simulink model "SmaSimulink"  (R2018a)
settings: Solver=FixedStepAuto  StartTime=0.0  StopTime=2  FixedStep=10e-6  RelTol=1e-6
values from neighbouring files (symbols this model uses):
  Af = 80 - ABS_ZERO_TEMP    (= 353.15)    [TempBris.m]    (also in TensileSMA.m = 353)
  As = 70 - ABS_ZERO_TEMP    (= 343.15)    [TempBris.m]    (also in TensileSMA.m = 343)
  Ca = 13.8 * 10^6    (= 13800000)    [TensileSMA.m]
  Cm = 8 * 10^6    (= 8000000)    [TensileSMA.m]
  cSf = 170 * 10^6    (= 170000000)    [TensileSMA.m]
  cSs = 100 * 10^6    (= 100000000)    [TensileSMA.m]
  Da = 6.7 * 10^4 * 10^6    (= 67000000000)    [TensileSMA.m]
  Dm = 2.63 * 10^4 * 10^6    (= 26300000000)    [TensileSMA.m]
  Mf = 40 - ABS_ZERO_TEMP    (= 313.15)    [TempBris.m]    (also in TensileSMA.m = 313)
  Ms = 50 - ABS_ZERO_TEMP    (= 323.15)    [TempBris.m]    (also in TensileSMA.m = 323)
  rEmax = 0.05    [TensileSMA.m]
undefined symbols (not defined in the file or in its folder): martDetwiningStrain, martDetwiningStress, sigma, simout, strain_mart, stress_mart, stressSweep, temp_mart_out
libraries: powerlib_meascontrol x1
(part 1 of 2)
settings Model: Creator=Michau  LastModifiedBy=Michau

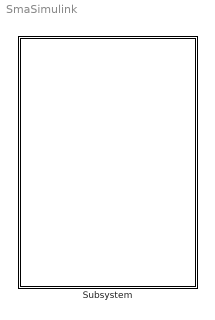
== system SmaSimulink ==
  Subsystem : Subsystem

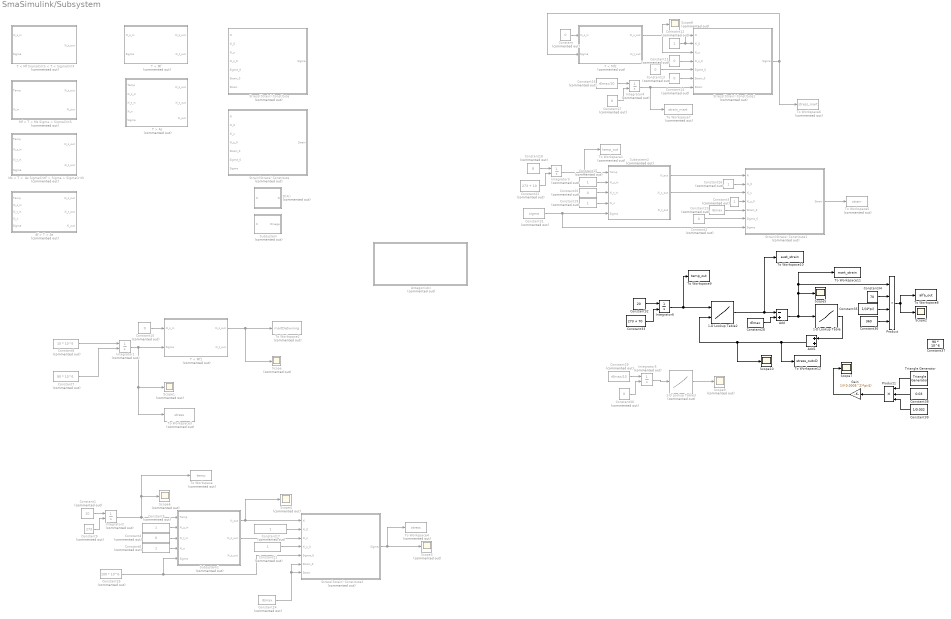
== system SmaSimulink/Subsystem ==
  1-D Lookup Table : Lookup_n-D  NumberOfTableDimensions=1  BreakpointsForDimension1=strain_mart  Table=stress_mart  InternalRulePriority=Speed  RndMeth=Simplest  InputSameDT=on
  1-D Lookup Table2 : Lookup_n-D  BreakpointsForDimension1=temp_mart_out  BreakpointsForDimension2=stressSweep  Table=simout  InternalRulePriority=Speed  RndMeth=Simplest  InputSameDT=on
  1-D Lookup Table3 : Lookup_n-D  Commented=on  NumberOfTableDimensions=1  BreakpointsForDimension1=strain_mart  Table=stress_mart  InternalRulePriority=Speed  RndMeth=Simplest  InputSameDT=on
  Add : Sum  Inputs=-+
  Add1 : Sum
  Af > T > As : Subsystem  Commented=on
  "Antagonistic " : Subsystem  Commented=on
  Constant{,2,4,10..11,13..14,20,27,30} (10 alike) : Constant  Commented=on  Value=0
  Constant1 : Constant  Commented=on  Value=10
  Constant{3,5..6,12,15,17,19,21,26} (9 alike) : Constant  Commented=on
  Constant16 : Constant  Commented=on  Value=rEmax/10
  Constant18 : Constant  Commented=on  Value=8
  Constant22 : Constant  Commented=on  Value=273 + 10
  Constant23 : Constant  Commented=on  Value=rEmax
  Constant24 : Constant  Commented=on  Value=rEmax
  Constant25 : Constant  Commented=on  Value=100 * 10^6
  Constant28 : Constant  Value=rEmax
  Constant29 : Constant  Commented=on  Value=rEmax/10
  Constant31 : Constant  Commented=on  Value=sigma
  Constant32 : Constant  Value=20
  Constant33 : Constant  Value=273 + 70
  Constant34 : Constant  Value=70
  Constant35 : Constant  Value=1/(4*pi)
  Constant36 : Constant  Value=360
  Constant37 : Constant  Value=90 * 10^6
  Constant38 : Constant  Value=0.03
  Constant39 : Constant  Value=1/0.002
  Constant7 : Constant  Commented=on  Value=90 * 10^6
  Constant8 : Constant  Commented=on  Value=10 * 10^6
  Constant9 : Constant  Commented=on  Value=273
  D(Xi) : Subsystem  Commented=on
  Gain : Gain  Gain=1/((0.0005^2)*pi/4)
  Integrator{1..5} (5 alike) : Integrator  Commented=on  InitialConditionSource=external
  Integrator6 : Integrator  InitialConditionSource=external
  Mf < T < Ms Sigma < SigmaCritS : Subsystem  Commented=on
  Ms < T <  As SigmaCritF > Sigma > SigmaCritS : Subsystem  Commented=on
  Product : Product  Inputs=4
  Product1 : Product  Inputs=3
  Scope{,1,3..4,6,8..9} (7 alike) : Scope  Commented=on
  Scope{2,5,7,10} (4 alike) : Scope
  Strain(Stress) Constitute : Subsystem  Commented=on
  Strain(Stress) Constitute1 : Subsystem  Commented=on
  Stress(Strain) Constitute : Subsystem  Commented=on
  Stress(Strain) Constitute1 : Subsystem  Commented=on
  Stress(Strain) Constitute2 : Subsystem  Commented=on
  Subsystem : Subsystem  Commented=on
  Subsystem1 : Subsystem  Commented=on
  Subsystem2 : Subsystem  Commented=on
  T < Mf : Subsystem  Commented=on
  T < Mf SigmaCritS < T < SigmaCritF : Subsystem  Commented=on
  T < Mf1 : Subsystem  Commented=on
  T < Mf2 : Subsystem  Commented=on
  T > As : Subsystem  Commented=on
  To Workspace : ToWorkspace  Commented=on  VariableName=temp  SampleTime=-1
  To Workspace1 : ToWorkspace  Commented=on  VariableName=temp_out  SampleTime=-1
  To Workspace10 : ToWorkspace  VariableName=aust_strain  SampleTime=-1
  To Workspace11 : ToWorkspace  VariableName=mart_strain  SampleTime=-1
  To Workspace12 : ToWorkspace  VariableName=stress_outxD  SampleTime=-1
  To Workspace2 : ToWorkspace  Commented=on  VariableName=martDetwining  SampleTime=-1
  To Workspace3 : ToWorkspace  Commented=on  VariableName=stress  SampleTime=-1
  To Workspace4 : ToWorkspace  Commented=on  VariableName=stress  SampleTime=-1
  To Workspace5 : ToWorkspace  Commented=on  VariableName=strain  SaveFormat=Timeseries  SampleTime=-1
  To Workspace6 : ToWorkspace  Commented=on  VariableName=stress_mart  SampleTime=-1
  To Workspace7 : ToWorkspace  Commented=on  VariableName=strain_mart  SampleTime=-1
  To Workspace8 : ToWorkspace  VariableName=alfa_out  SampleTime=-1
  To Workspace9 : ToWorkspace  VariableName=temp_out  SampleTime=-1
  Triangle Generator : powerlib_meascontrol/Pulse & Signal Generators/Triangle Generator  Freq=1/4  Phase=90  Ts=0
  wires:
  Constant18/1 -> Integrator3/1
  Constant22/1 -> Integrator3/2
  Constant26/1 -> Strain(Stress) Constitute1/2(Xi_0)
  Constant3/1 -> Strain(Stress) Constitute1/4(Xi_s_0)
  ? -> Stress(Strain) Constitute/5(Sigma_0)
  Strain(Stress) Constitute1/1(Strain) -> To Workspace5/1
  Constant5/1 -> Subsystem1/2(Xi_s_in)
  Constant6/1 -> Subsystem1/4(Xi_n)
  Constant9/1 -> Integrator2/2
  Integrator2/1 -> To Workspace/1, Scope6/1, Subsystem1/1(Temp)
  Constant1/1 -> Integrator2/1
  Constant4/1 -> Subsystem1/3(Xi_t_in)
  Constant17/1 -> Stress(Strain) Constitute2/2(Xi_0)
  Subsystem1/1(Xi_out) -> Scope4/1, Stress(Strain) Constitute2/1(Xi)
  Constant21/1 -> Stress(Strain) Constitute2/4(Xi_s_0)
  Subsystem1/2(Xi_s_out) -> Stress(Strain) Constitute2/3(Xi_s)
  Constant24/1 -> Stress(Strain) Constitute2/6(Strain_0), Stress(Strain) Constitute2/7(Strain)
  Constant25/1 -> Subsystem1/5(Sigma), Stress(Strain) Constitute2/5(Sigma_0)
  Stress(Strain) Constitute2/1(Sigma) -> To Workspace4/1, Scope3/1
  Integrator1/1 -> T < Mf1/2(Sigma), Scope1/1, To Workspace3/1
  Constant10/1 -> T < Mf1/1(Xi_s_in)
  T < Mf1/1(Xi_s_out) -> Scope/1, To Workspace2/1
  Constant7/1 -> Integrator1/2
  Constant8/1 -> Integrator1/1
  T < Mf2/1(Xi_s_out) -> Scope8/1, Stress(Strain) Constitute1/3(Xi_s)
  Constant/1 -> T < Mf2/1(Xi_s_in)
  Constant11/1 -> Stress(Strain) Constitute1/4(Xi_s_0)
  Constant12/1 -> Stress(Strain) Constitute1/1(Xi), Stress(Strain) Constitute1/2(Xi_0)
  Constant13/1 -> Stress(Strain) Constitute1/5(Sigma_0)
  Constant14/1 -> Stress(Strain) Constitute1/6(Strain_0)
  Integrator4/1 -> To Workspace7/1, Stress(Strain) Constitute1/7(Strain)
  Constant27/1 -> Integrator4/2
  Constant16/1 -> Integrator4/1
  Stress(Strain) Constitute1/1(Sigma) -> T < Mf2/2(Sigma), To Workspace6/1
  Subsystem2/1(Xi_out) -> Strain(Stress) Constitute1/1(Xi)
  Subsystem2/2(Xi_s_out) -> Strain(Stress) Constitute1/3(Xi_s)
  Integrator3/1 -> To Workspace1/1, Subsystem2/1(Temp)
  Constant15/1 -> Subsystem2/2(Xi_s_in)
  Constant19/1 -> Subsystem2/4(Xi_n)
  Constant20/1 -> Subsystem2/3(Xi_t_in)
  Constant23/1 -> Strain(Stress) Constitute1/5(Strain_0)
  Constant2/1 -> Strain(Stress) Constitute1/6(Sigma_0)
  Constant28/1 -> Add/2
  Add/1 -> Scope5/1, To Workspace11/1, Product/1, 1-D Lookup Table/1
  Constant30/1 -> Integrator5/2
  Integrator5/1 -> 1-D Lookup Table3/1
  Constant29/1 -> Integrator5/1
  1-D Lookup Table3/1 -> Scope9/1
  Constant31/1 -> Strain(Stress) Constitute1/7(Sigma), Subsystem2/5(Sigma)
  Constant33/1 -> Integrator6/2
  Constant32/1 -> Integrator6/1
  Integrator6/1 -> To Workspace9/1, 1-D Lookup Table2/1
  1-D Lookup Table2/1 -> To Workspace10/1, Add/1
  Constant34/1 -> Product/2
  Constant35/1 -> Product/3
  Product/1 -> To Workspace8/1, Scope2/1
  Constant36/1 -> Product/4
  1-D Lookup Table/1 -> Add1/1
  Add1/1 -> To Workspace12/1, Scope10/1, 1-D Lookup Table2/2
  Triangle Generator/1 -> Product1/1
  Constant38/1 -> Product1/2
  Constant39/1 -> Product1/3
  Product1/1 -> Gain/1
  Gain/1 -> Scope7/1

== system SmaSimulink/Subsystem/Af > T > As ==
  Temp : Inport
  Xi_s_in : Inport  Port=2
  Xi_t_in : Inport  Port=3
  Xi_n : Inport  Port=4
  Sigma : Inport  Port=5
  "T > As Xi " : Subsystem
  T > As Xi_s : Subsystem
  T > As Xi_t : Subsystem
  Xi_s_out : Outport
  Xi_t_out : Outport  Port=2
  Xi_out : Outport  Port=3
  wires:
  Sigma/1 -> "T > As Xi "/3("Sigma ")
  "T > As Xi "/1(Xi_out) -> T > As Xi_s/3(Xi_out), T > As Xi_t/3(Xi_out), Xi_out/1
  Xi_s_in/1 -> T > As Xi_s/1("Xi_s_in ")
  Xi_n/1 -> "T > As Xi "/1(Xi_in), T > As Xi_t/2(Xi_in), T > As Xi_s/2(Xi_in)
  T > As Xi_s/1(Xi_s_out) -> Xi_s_out/1
  Temp/1 -> "T > As Xi "/2(T)
  Xi_t_in/1 -> T > As Xi_t/1("Xi_t_in ")
  T > As Xi_t/1(Xi_t_out) -> Xi_t_out/1

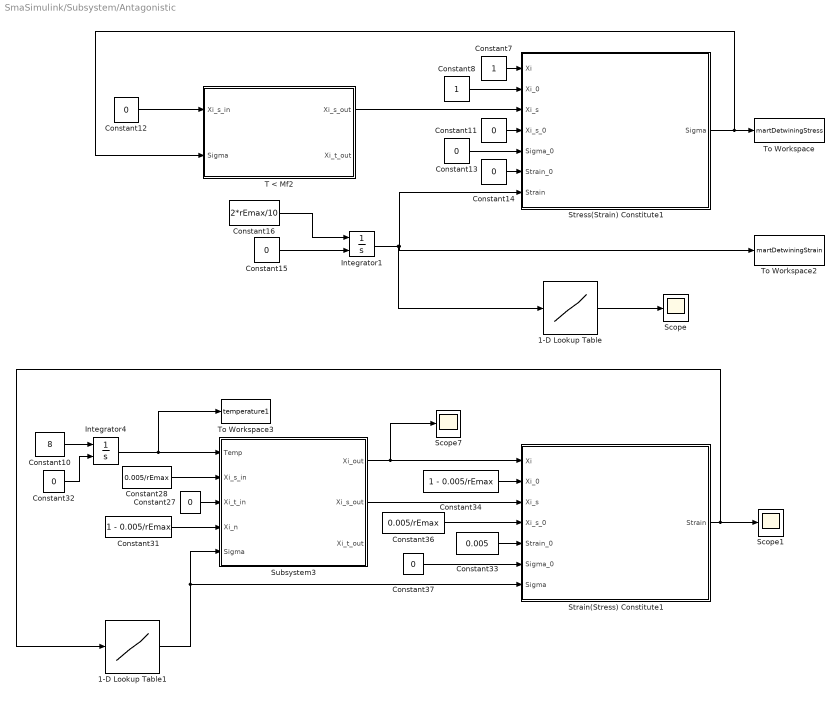
== system SmaSimulink/Subsystem/Antagonistic  ==
  1-D Lookup Table : Lookup_n-D  NumberOfTableDimensions=1  BreakpointsForDimension1=martDetwiningStrain  Table=martDetwiningStress  InternalRulePriority=Speed  RndMeth=Simplest  InputSameDT=on
  1-D Lookup Table1 : Lookup_n-D  NumberOfTableDimensions=1  BreakpointsForDimension1=martDetwiningStrain  Table=martDetwiningStress  InternalRulePriority=Speed  RndMeth=Simplest  InputSameDT=on
  Constant10 : Constant  Value=8
  Constant{11..15,27,32,37} (8 alike) : Constant  Value=0
  Constant16 : Constant  Value=2*rEmax/10
  Constant28 : Constant  Value=0.005/rEmax
  Constant31 : Constant  Value=1 - 0.005/rEmax
  Constant33 : Constant  Value=0.005
  Constant34 : Constant  Value=1 - 0.005/rEmax
  Constant36 : Constant  Value=0.005/rEmax
  Constant7 : Constant
  Constant8 : Constant
  Integrator1 : Integrator  InitialConditionSource=external
  Integrator4 : Integrator  InitialConditionSource=external
  Scope : Scope
  Scope1 : Scope
  Scope7 : Scope
  Strain(Stress) Constitute1 : Subsystem
  Stress(Strain) Constitute1 : Subsystem
  Subsystem3 : Subsystem
  T < Mf2 : Subsystem
  To Workspace : ToWorkspace  VariableName=martDetwiningStress  SampleTime=-1
  To Workspace2 : ToWorkspace  VariableName=martDetwiningStrain  SampleTime=-1
  To Workspace3 : ToWorkspace  VariableName=temperature1  SampleTime=-1
  wires:
  Constant7/1 -> Stress(Strain) Constitute1/1(Xi)
  Stress(Strain) Constitute1/1(Sigma) -> To Workspace/1, T < Mf2/2(Sigma)
  Constant28/1 -> Subsystem3/2(Xi_s_in)
  Constant8/1 -> Stress(Strain) Constitute1/2(Xi_0)
  Constant12/1 -> T < Mf2/1(Xi_s_in)
  Constant34/1 -> Strain(Stress) Constitute1/2(Xi_0)
  Constant16/1 -> Integrator1/1
  Strain(Stress) Constitute1/1(Strain) -> Scope1/1, 1-D Lookup Table1/1
  Integrator4/1 -> To Workspace3/1, Subsystem3/1(Temp)
  Integrator1/1 -> 1-D Lookup Table/1, To Workspace2/1, Stress(Strain) Constitute1/7(Strain)
  Constant14/1 -> Stress(Strain) Constitute1/6(Strain_0)
  T < Mf2/1(Xi_s_out) -> Stress(Strain) Constitute1/3(Xi_s)
  Subsystem3/1(Xi_out) -> Scope7/1, Strain(Stress) Constitute1/1(Xi)
  1-D Lookup Table/1 -> Scope/1
  Constant15/1 -> Integrator1/2
  Constant37/1 -> Strain(Stress) Constitute1/6(Sigma_0)
  Constant33/1 -> Strain(Stress) Constitute1/5(Strain_0)
  Constant32/1 -> Integrator4/2
  Constant31/1 -> Subsystem3/4(Xi_n)
  Constant11/1 -> Stress(Strain) Constitute1/4(Xi_s_0)
  Constant36/1 -> Strain(Stress) Constitute1/4(Xi_s_0)
  Constant10/1 -> Integrator4/1
  Subsystem3/2(Xi_s_out) -> Strain(Stress) Constitute1/3(Xi_s)
  1-D Lookup Table1/1 -> Strain(Stress) Constitute1/7(Sigma), Subsystem3/5(Sigma)
  Constant13/1 -> Stress(Strain) Constitute1/5(Sigma_0)
  Constant27/1 -> Subsystem3/3(Xi_t_in)

== system SmaSimulink/Subsystem/D(Xi) ==
  Xi : Inport
  Add : Sum
  Constant : Constant  Value=Dm-Da
  Constant1 : Constant  Value=Da
  Product : Product
  D : Outport
  wires:
  Xi/1 -> Product/2
  Product/1 -> Add/1
  Constant1/1 -> Add/2
  Constant/1 -> Product/1
  Add/1 -> D/1

== system SmaSimulink/Subsystem/Mf < T < Ms Sigma < SigmaCritS ==
  Temp : Inport
  Xi_in : Inport  Port=2
  Add : Sum  Inputs=-+
  Add1 : Sum  Inputs=+-
  Add2 : Sum
  Constant : Constant
  Constant1 : Constant
  Constant2 : Constant  Value=pi/(Ms-Mf)
  Constant4 : Constant  Value=Mf
  Cos1 : Trigonometry  Operator=cos
  Product1 : Product
  Product3 : Product
  "[(1-x)/2]" : Subsystem
  "Xi_t_out " : Outport
  Xi_out : Outport  Port=2
  wires:
  "[(1-x)/2]"/1(Out) -> Product1/2
  Constant1/1 -> Add2/1
  Xi_in/1 -> "[(1-x)/2]"/1(In)
  Product3/1 -> Cos1/1
  Temp/1 -> Add1/1
  Add1/1 -> Product3/2
  Add2/1 -> Product1/1
  Constant2/1 -> Product3/1
  Cos1/1 -> Add2/2
  Constant4/1 -> Add1/2
  Constant/1 -> Add/2
  Product1/1 -> "Xi_t_out "/1, Add/1
  Add/1 -> Xi_out/1

== system SmaSimulink/Subsystem/Ms < T <  As SigmaCritF > Sigma > SigmaCritS ==
  Temp : Inport
  Xi_s_in : Inport  Port=2
  Xi_t_in : Inport  Port=3
  Sigma : Inport  Port=4
  T > Ms Xi_s : Subsystem
  T > Ms Xi_t : Subsystem
  Xi_s_out : Outport
  Xi_t_out : Outport  Port=2
  wires:
  Sigma/1 -> T > Ms Xi_s/2(Sigma)
  Temp/1 -> T > Ms Xi_s/3(Temp)
  Xi_s_in/1 -> T > Ms Xi_t/2(Xi_s_in), T > Ms Xi_s/1(Xi_s_in)
  Xi_t_in/1 -> T > Ms Xi_t/1(Xi_t_in)
  T > Ms Xi_s/1(Xi_s_out) -> T > Ms Xi_t/3(Xi_s_out), Xi_s_out/1
  T > Ms Xi_t/1(Xi_t_out) -> Xi_t_out/1

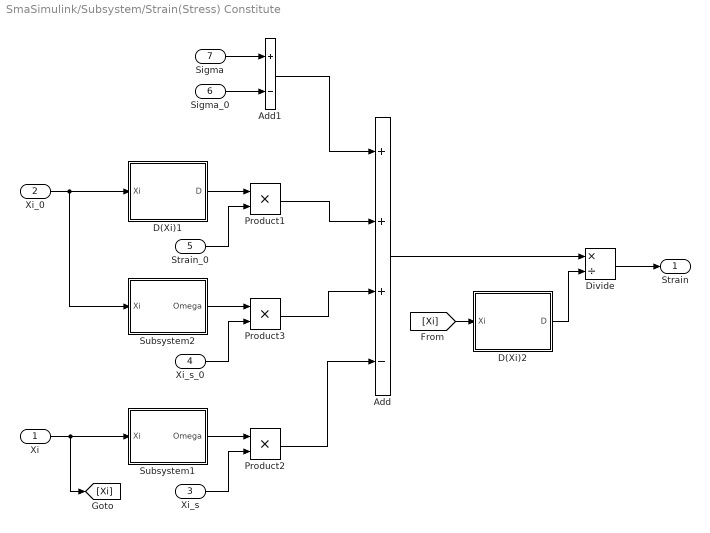
== system SmaSimulink/Subsystem/Strain(Stress) Constitute ==
  Xi : Inport
  Xi_0 : Inport  Port=2
  Xi_s : Inport  Port=3
  Xi_s_0 : Inport  Port=4
  Strain_0 : Inport  Port=5
  Sigma_0 : Inport  Port=6
  Sigma : Inport  Port=7
  Add : Sum  Inputs=+++-
  Add1 : Sum  Inputs=+-
  D(Xi)1 : Subsystem
  D(Xi)2 : Subsystem
  Divide : Product  Inputs=*/
  Product1 : Product
  Product2 : Product
  Product3 : Product
  Subsystem1 : Subsystem
  Subsystem2 : Subsystem
  Strain : Outport
  wires:
  D(Xi)1/1(D) -> Product1/1
  Strain_0/1 -> Product1/2
  Xi/1 -> Subsystem1/1(Xi), [Xi]
  Subsystem1/1(Omega) -> Product2/1
  Xi_0/1 -> Subsystem2/1(Xi), D(Xi)1/1(Xi)
  Subsystem2/1(Omega) -> Product3/1
  Xi_s_0/1 -> Product3/2
  Add/1 -> Divide/1
  Sigma_0/1 -> Add1/2
  Sigma/1 -> Add1/1
  Add1/1 -> Add/1
  Xi_s/1 -> Product2/2
  Product1/1 -> Add/2
  Product3/1 -> Add/3
  Product2/1 -> Add/4
  [Xi] -> D(Xi)2/1(Xi)
  D(Xi)2/1(D) -> Divide/2
  Divide/1 -> Strain/1

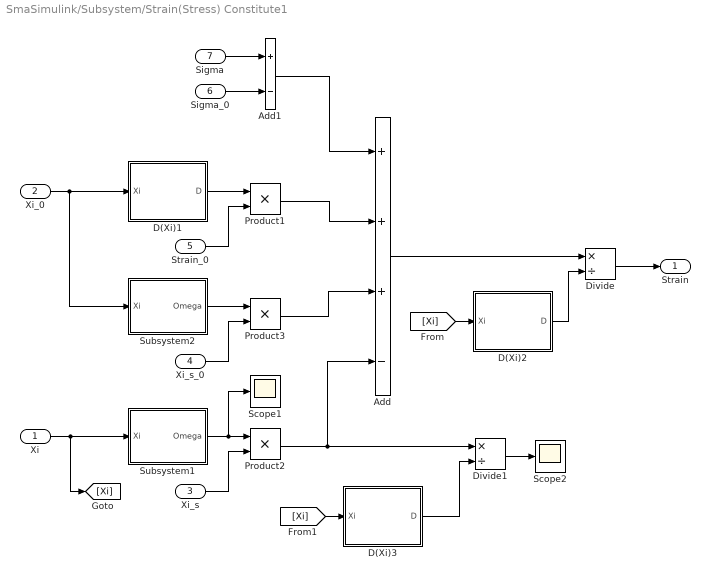
== system SmaSimulink/Subsystem/Strain(Stress) Constitute1 ==
  Xi : Inport
  Xi_0 : Inport  Port=2
  Xi_s : Inport  Port=3
  Xi_s_0 : Inport  Port=4
  Strain_0 : Inport  Port=5
  Sigma_0 : Inport  Port=6
  Sigma : Inport  Port=7
  Add : Sum  Inputs=+++-
  Add1 : Sum  Inputs=+-
  D(Xi)1 : Subsystem
  D(Xi)2 : Subsystem
  D(Xi)3 : Subsystem
  Divide : Product  Inputs=*/
  Divide1 : Product  Inputs=*/
  Product1 : Product
  Product2 : Product
  Product3 : Product
  Scope1 : Scope
  Scope2 : Scope
  Subsystem1 : Subsystem
  Subsystem2 : Subsystem
  Strain : Outport
  wires:
  D(Xi)1/1(D) -> Product1/1
  Strain_0/1 -> Product1/2
  Xi/1 -> Subsystem1/1(Xi), [Xi]
  Subsystem1/1(Omega) -> Scope1/1, Product2/1
  Xi_0/1 -> Subsystem2/1(Xi), D(Xi)1/1(Xi)
  Subsystem2/1(Omega) -> Product3/1
  Xi_s_0/1 -> Product3/2
  Add/1 -> Divide/1
  Sigma_0/1 -> Add1/2
  Sigma/1 -> Add1/1
  Add1/1 -> Add/1
  Xi_s/1 -> Product2/2
  Product1/1 -> Add/2
  Product3/1 -> Add/3
  Product2/1 -> Add/4, Divide1/1
  [Xi] -> D(Xi)2/1(Xi)
  D(Xi)2/1(D) -> Divide/2
  Divide/1 -> Strain/1
  [Xi] -> D(Xi)3/1(Xi)
  D(Xi)3/1(D) -> Divide1/2
  Divide1/1 -> Scope2/1

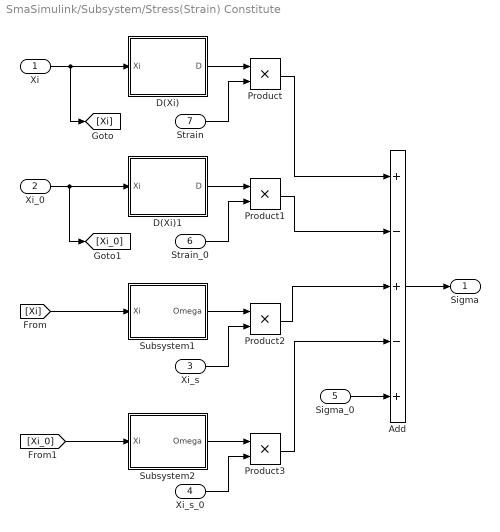
== system SmaSimulink/Subsystem/Stress(Strain) Constitute ==
  Xi : Inport
  Xi_0 : Inport  Port=2
  Xi_s : Inport  Port=3
  Xi_s_0 : Inport  Port=4
  Sigma_0 : Inport  Port=5
  Strain_0 : Inport  Port=6
  Strain : Inport  Port=7
  Add : Sum  Inputs=+-+-+
  D(Xi) : Subsystem
  D(Xi)1 : Subsystem
  Product{,1..3} (4 alike) : Product
  Subsystem1 : Subsystem
  Subsystem2 : Subsystem
  Sigma : Outport
  wires:
  Xi/1 -> [Xi], D(Xi)/1(Xi)
  D(Xi)/1(D) -> Product/1
  Strain/1 -> Product/2
  Xi_0/1 -> [Xi_0], D(Xi)1/1(Xi)
  D(Xi)1/1(D) -> Product1/1
  Strain_0/1 -> Product1/2
  [Xi] -> Subsystem1/1(Xi)
  Subsystem1/1(Omega) -> Product2/1
  Xi_s/1 -> Product2/2
  [Xi_0] -> Subsystem2/1(Xi)
  Subsystem2/1(Omega) -> Product3/1
  Xi_s_0/1 -> Product3/2
  Product/1 -> Add/1
  Product1/1 -> Add/2
  Product2/1 -> Add/3
  Product3/1 -> Add/4
  Sigma_0/1 -> Add/5
  Add/1 -> Sigma/1

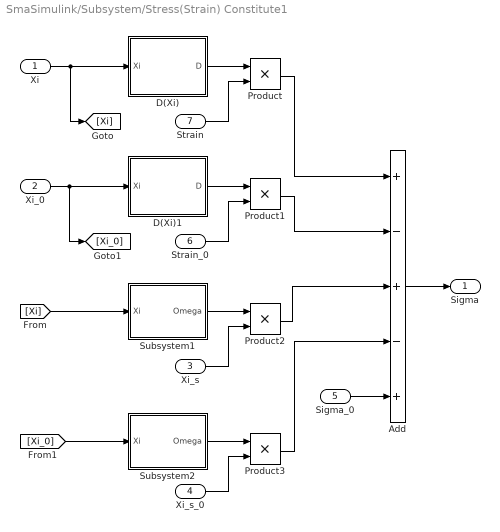
== system SmaSimulink/Subsystem/Stress(Strain) Constitute1 ==
  Xi : Inport
  Xi_0 : Inport  Port=2
  Xi_s : Inport  Port=3
  Xi_s_0 : Inport  Port=4
  Sigma_0 : Inport  Port=5
  Strain_0 : Inport  Port=6
  Strain : Inport  Port=7
  Add : Sum  Inputs=+-+-+
  D(Xi) : Subsystem
  D(Xi)1 : Subsystem
  Product{,1..3} (4 alike) : Product
  Subsystem1 : Subsystem
  Subsystem2 : Subsystem
  Sigma : Outport
  wires:
  Xi/1 -> [Xi], D(Xi)/1(Xi)
  D(Xi)/1(D) -> Product/1
  Strain/1 -> Product/2
  Xi_0/1 -> [Xi_0], D(Xi)1/1(Xi)
  D(Xi)1/1(D) -> Product1/1
  Strain_0/1 -> Product1/2
  [Xi] -> Subsystem1/1(Xi)
  Subsystem1/1(Omega) -> Product2/1
  Xi_s/1 -> Product2/2
  [Xi_0] -> Subsystem2/1(Xi)
  Subsystem2/1(Omega) -> Product3/1
  Xi_s_0/1 -> Product3/2
  Product/1 -> Add/1
  Product1/1 -> Add/2
  Product2/1 -> Add/3
  Product3/1 -> Add/4
  Sigma_0/1 -> Add/5
  Add/1 -> Sigma/1

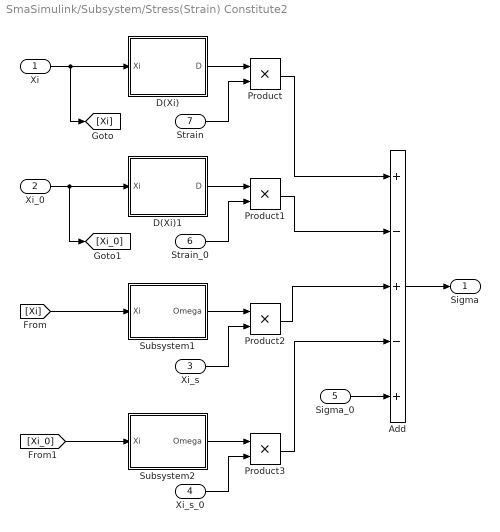
== system SmaSimulink/Subsystem/Stress(Strain) Constitute2 ==
  Xi : Inport
  Xi_0 : Inport  Port=2
  Xi_s : Inport  Port=3
  Xi_s_0 : Inport  Port=4
  Sigma_0 : Inport  Port=5
  Strain_0 : Inport  Port=6
  Strain : Inport  Port=7
  Add : Sum  Inputs=+-+-+
  D(Xi) : Subsystem
  D(Xi)1 : Subsystem
  Product{,1..3} (4 alike) : Product
  Subsystem1 : Subsystem
  Subsystem2 : Subsystem
  Sigma : Outport
  wires:
  Xi/1 -> [Xi], D(Xi)/1(Xi)
  D(Xi)/1(D) -> Product/1
  Strain/1 -> Product/2
  Xi_0/1 -> [Xi_0], D(Xi)1/1(Xi)
  D(Xi)1/1(D) -> Product1/1
  Strain_0/1 -> Product1/2
  [Xi] -> Subsystem1/1(Xi)
  Subsystem1/1(Omega) -> Product2/1
  Xi_s/1 -> Product2/2
  [Xi_0] -> Subsystem2/1(Xi)
  Subsystem2/1(Omega) -> Product3/1
  Xi_s_0/1 -> Product3/2
  Product/1 -> Add/1
  Product1/1 -> Add/2
  Product2/1 -> Add/3
  Product3/1 -> Add/4
  Sigma_0/1 -> Add/5
  Add/1 -> Sigma/1

== system SmaSimulink/Subsystem/Subsystem ==
  Xi : Inport
  Constant : Constant  Value=-rEmax
  Product : Product
  Subsystem1 : Subsystem
  Omega : Outport
  wires:
  Product/1 -> Omega/1
  Subsystem1/1(D) -> Product/1
  Constant/1 -> Product/2
  Xi/1 -> Subsystem1/1(Xi)

== system SmaSimulink/Subsystem/Subsystem1 ==
  Temp : Inport
  Xi_s_in : Inport  Port=2
  Xi_t_in : Inport  Port=3
  Xi_n : Inport  Port=4
  Sigma : Inport  Port=5
  Af > T > As1 : Subsystem
  Demux : Demux  Outputs=3
  Memory : Memory
  Mux : Mux  Inputs=3
  Mux2 : Mux  Inputs=3
  Range check : Subsystem
  Xi_out : Outport
  Xi_s_out : Outport  Port=2
  Xi_t_out : Outport  Port=3
  wires:
  Af > T > As1/2(Xi_t_out) -> Mux/2
  Af > T > As1/3(Xi_out) -> Mux/3
  Sigma/1 -> Memory/1, Af > T > As1/5(Sigma)
  Temp/1 -> Range check/1(T), Af > T > As1/1(Temp)
  Xi_n/1 -> Mux2/3, Af > T > As1/4(Xi_n)
  Xi_s_in/1 -> Mux2/1, Af > T > As1/2(Xi_s_in)
  Xi_t_in/1 -> Mux2/2, Af > T > As1/3(Xi_t_in)
  Af > T > As1/1(Xi_s_out) -> Mux/1
  Demux/1 -> Xi_s_out/1
  Demux/2 -> Xi_t_out/1
  Demux/3 -> Xi_out/1
  Mux/1 -> Range check/2(Xis_new)
  Mux2/1 -> Range check/3(Xis_old)
  Range check/1(Out1) -> Demux/1
  Memory/1 -> Range check/4(Stress)

== system SmaSimulink/Subsystem/Subsystem2 ==
  Temp : Inport
  Xi_s_in : Inport  Port=2
  Xi_t_in : Inport  Port=3
  Xi_n : Inport  Port=4
  Sigma : Inport  Port=5
  Af > T > As1 : Subsystem
  Demux : Demux  Outputs=3
  Memory : Memory
  Mux : Mux  Inputs=3
  Mux2 : Mux  Inputs=3
  Range check : Subsystem
  Xi_out : Outport
  Xi_s_out : Outport  Port=2
  Xi_t_out : Outport  Port=3
  wires:
  Af > T > As1/2(Xi_t_out) -> Mux/2
  Af > T > As1/3(Xi_out) -> Mux/3
  Sigma/1 -> Memory/1, Af > T > As1/5(Sigma)
  Temp/1 -> Range check/1(T), Af > T > As1/1(Temp)
  Xi_n/1 -> Mux2/3, Af > T > As1/4(Xi_n)
  Xi_s_in/1 -> Mux2/1, Af > T > As1/2(Xi_s_in)
  Xi_t_in/1 -> Mux2/2, Af > T > As1/3(Xi_t_in)
  Af > T > As1/1(Xi_s_out) -> Mux/1
  Demux/1 -> Xi_s_out/1
  Demux/2 -> Xi_t_out/1
  Demux/3 -> Xi_out/1
  Mux/1 -> Range check/2(Xis_new)
  Mux2/1 -> Range check/3(Xis_old)
  Range check/1(Out1) -> Demux/1
  Memory/1 -> Range check/4(Stress)

== system SmaSimulink/Subsystem/T < Mf ==
  Xi_s_in : Inport
  Sigma : Inport  Port=2
  Add : Sum  Inputs=-+
  Constant3 : Constant  Value=0
  Constant4 : Constant
  Constant5 : Constant
  Switch : Switch  Criteria=u2 > Threshold  Threshold=cSs
  Switch1 : Switch  Criteria=u2 > Threshold  Threshold=cSf
  T < Mf SigmaCritS < T < SigmaCritF : Subsystem
  Xi_s_out : Outport
  "Xi_t_out " : Outport  Port=2
  wires:
  Constant3/1 -> Switch/3
  Sigma/1 -> Switch/2, Switch1/2, T < Mf SigmaCritS < T < SigmaCritF/2(Sigma)
  Switch/1 -> Switch1/3
  T < Mf SigmaCritS < T < SigmaCritF/1(Xi_t_out) -> Switch/1
  Xi_s_in/1 -> T < Mf SigmaCritS < T < SigmaCritF/1(Xi_s_in)
  Constant4/1 -> Add/2
  Switch1/1 -> Xi_s_out/1, Add/1
  Constant5/1 -> Switch1/1
  Add/1 -> "Xi_t_out "/1

== system SmaSimulink/Subsystem/T < Mf SigmaCritS < T < SigmaCritF ==
  Xi_s_in : Inport
  Sigma : Inport  Port=2
  Add1 : Sum  Inputs=+-
  Add3 : Sum
  Constant1 : Constant  Value=cSf
  Constant2 : Constant  Value=pi/(cSs-cSf)
  Cos : Trigonometry  Operator=cos
  Product2 : Product
  Product3 : Product
  "[(1+x)/2]" : Subsystem
  "[(1-x)/2]" : Subsystem
  Xi_t_out : Outport
  wires:
  Cos/1 -> Product2/2
  Product2/1 -> Add3/2
  Add1/1 -> Product3/2
  Sigma/1 -> Add1/1
  Add3/1 -> Xi_t_out/1
  Xi_s_in/1 -> "[(1+x)/2]"/1(In), "[(1-x)/2]"/1(In)
  Product3/1 -> Cos/1
  "[(1+x)/2]"/1(Out) -> Add3/1
  "[(1-x)/2]"/1(Out) -> Product2/1
  Constant2/1 -> Product3/1
  Constant1/1 -> Add1/2

== system SmaSimulink/Subsystem/T < Mf1 ==
  Xi_s_in : Inport
  Sigma : Inport  Port=2
  Add : Sum  Inputs=-+
  Constant3 : Constant  Value=0
  Constant4 : Constant
  Constant5 : Constant
  Switch : Switch  Criteria=u2 > Threshold  Threshold=cSs
  Switch1 : Switch  Criteria=u2 > Threshold  Threshold=cSf
  T < Mf SigmaCritS < T < SigmaCritF : Subsystem
  Xi_s_out : Outport
  "Xi_t_out " : Outport  Port=2
  wires:
  Constant3/1 -> Switch/3
  Sigma/1 -> Switch/2, Switch1/2, T < Mf SigmaCritS < T < SigmaCritF/2(Sigma)
  Switch/1 -> Switch1/3
  T < Mf SigmaCritS < T < SigmaCritF/1(Xi_t_out) -> Switch/1
  Xi_s_in/1 -> T < Mf SigmaCritS < T < SigmaCritF/1(Xi_s_in)
  Constant4/1 -> Add/2
  Switch1/1 -> Xi_s_out/1, Add/1
  Constant5/1 -> Switch1/1
  Add/1 -> "Xi_t_out "/1

== system SmaSimulink/Subsystem/T < Mf2 ==
  Xi_s_in : Inport
  Sigma : Inport  Port=2
  Add : Sum  Inputs=-+
  Constant3 : Constant  Value=0
  Constant4 : Constant
  Constant5 : Constant
  Switch : Switch  Criteria=u2 > Threshold  Threshold=cSs
  Switch1 : Switch  Criteria=u2 > Threshold  Threshold=cSf
  T < Mf SigmaCritS < T < SigmaCritF : Subsystem
  Xi_s_out : Outport
  "Xi_t_out " : Outport  Port=2
  wires:
  Constant3/1 -> Switch/3
  Sigma/1 -> Switch/2, Switch1/2, T < Mf SigmaCritS < T < SigmaCritF/2(Sigma)
  Switch/1 -> Switch1/3
  T < Mf SigmaCritS < T < SigmaCritF/1(Xi_t_out) -> Switch/1
  Xi_s_in/1 -> T < Mf SigmaCritS < T < SigmaCritF/1(Xi_s_in)
  Constant4/1 -> Add/2
  Switch1/1 -> Xi_s_out/1, Add/1
  Constant5/1 -> Switch1/1
  Add/1 -> "Xi_t_out "/1

== system SmaSimulink/Subsystem/T > As ==
  Temp : Inport
  Xi_s_in : Inport  Port=2
  Xi_t_in : Inport  Port=3
  Xi_n : Inport  Port=4
  Sigma : Inport  Port=5
  Af > T > As1 : Subsystem
  Constant3 : Constant  Value=[0 0 0]
  Demux : Demux  Outputs=3
  Mux : Mux  Inputs=3
  Mux2 : Mux  Inputs=3
  Switch : Switch  Criteria=u2 > Threshold  Threshold=As
  Switch1 : Switch  Criteria=u2 > Threshold  Threshold=Af
  Xi_s_out : Outport
  Xi_t_out : Outport  Port=2
  Xi_out : Outport  Port=3
  wires:
  Constant3/1 -> Switch1/1
  Mux2/1 -> Switch/3
  Af > T > As1/2(Xi_t_out) -> Mux/2
  Switch/1 -> Switch1/3
  Af > T > As1/3(Xi_out) -> Mux/3
  Sigma/1 -> Af > T > As1/5(Sigma)
  Temp/1 -> Switch1/2, Switch/2, Af > T > As1/1(Temp)
  Xi_n/1 -> Mux2/3, Af > T > As1/4(Xi_n)
  Xi_s_in/1 -> Mux2/1, Af > T > As1/2(Xi_s_in)
  Xi_t_in/1 -> Mux2/2, Af > T > As1/3(Xi_t_in)
  Af > T > As1/1(Xi_s_out) -> Mux/1
  Mux/1 -> Switch/1
  Switch1/1 -> Demux/1
  Demux/1 -> Xi_s_out/1
  Demux/2 -> Xi_t_out/1
  Demux/3 -> Xi_out/1

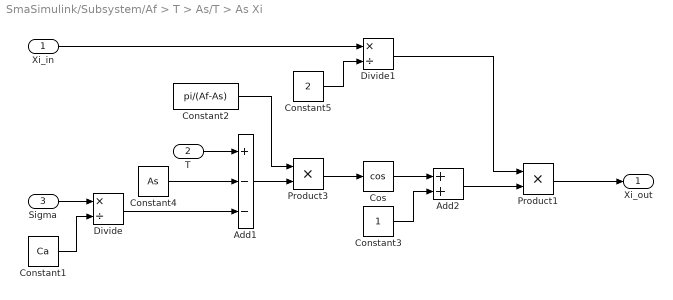
== system SmaSimulink/Subsystem/Af > T > As/T > As Xi  ==
  Xi_in : Inport
  T : Inport  Port=2
  "Sigma " : Inport  Port=3
  Add1 : Sum  Inputs=+--
  Add2 : Sum
  Constant1 : Constant  Value=Ca
  Constant2 : Constant  Value=pi/(Af-As)
  Constant3 : Constant
  Constant4 : Constant  Value=As
  Constant5 : Constant  Value=2
  Cos : Trigonometry  Operator=cos
  Divide : Product  Inputs=*/
  Divide1 : Product  Inputs=*/
  Product1 : Product
  Product3 : Product
  Xi_out : Outport
  wires:
  Constant4/1 -> Add1/2
  Xi_in/1 -> Divide1/1
  T/1 -> Add1/1
  Add1/1 -> Product3/2
  Constant2/1 -> Product3/1
  Product3/1 -> Cos/1
  "Sigma "/1 -> Divide/1
  Constant1/1 -> Divide/2
  Divide/1 -> Add1/3
  Cos/1 -> Add2/1
  Constant3/1 -> Add2/2
  Constant5/1 -> Divide1/2
  Add2/1 -> Product1/2
  Divide1/1 -> Product1/1
  Product1/1 -> Xi_out/1

== system SmaSimulink/Subsystem/Af > T > As/T > As Xi_s ==
  "Xi_s_in " : Inport
  Xi_in : Inport  Port=2
  Xi_out : Inport  Port=3
  Add1 : Sum  Inputs=+-
  Add2 : Sum  Inputs=+-
  Divide : Product  Inputs=*/
  Product1 : Product
  Xi_s_out : Outport
  wires:
  Xi_in/1 -> Add2/1, Divide/2
  "Xi_s_in "/1 -> Add1/1, Divide/1
  Add1/1 -> Xi_s_out/1
  Xi_out/1 -> Add2/2
  Divide/1 -> Product1/1
  Add2/1 -> Product1/2
  Product1/1 -> Add1/2

== system SmaSimulink/Subsystem/Af > T > As/T > As Xi_t ==
  "Xi_t_in " : Inport
  Xi_in : Inport  Port=2
  Xi_out : Inport  Port=3
  Add1 : Sum  Inputs=+-
  Add2 : Sum  Inputs=+-
  Divide : Product  Inputs=*/
  Product1 : Product
  Xi_t_out : Outport
  wires:
  Xi_in/1 -> Add2/1, Divide/2
  "Xi_t_in "/1 -> Add1/1, Divide/1
  Add1/1 -> Xi_t_out/1
  Xi_out/1 -> Add2/2
  Divide/1 -> Product1/1
  Add2/1 -> Product1/2
  Product1/1 -> Add1/2

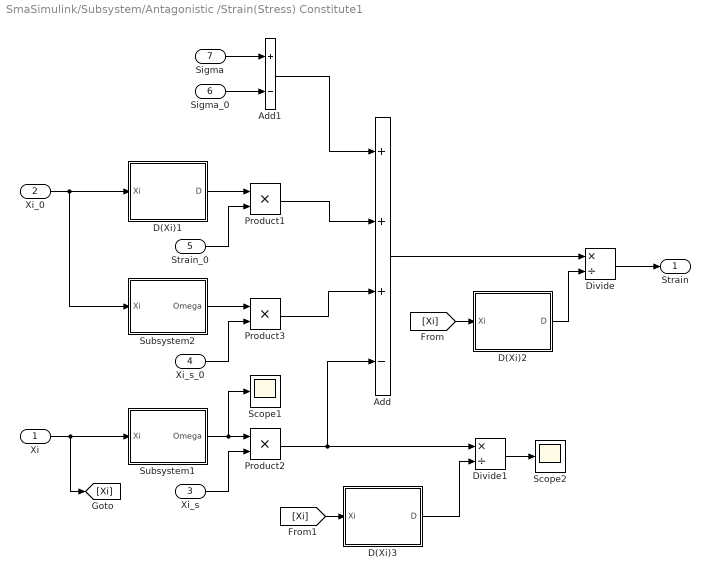
== system SmaSimulink/Subsystem/Antagonistic /Strain(Stress) Constitute1 ==
  Xi : Inport
  Xi_0 : Inport  Port=2
  Xi_s : Inport  Port=3
  Xi_s_0 : Inport  Port=4
  Strain_0 : Inport  Port=5
  Sigma_0 : Inport  Port=6
  Sigma : Inport  Port=7
  Add : Sum  Inputs=+++-
  Add1 : Sum  Inputs=+-
  D(Xi)1 : Subsystem
  D(Xi)2 : Subsystem
  D(Xi)3 : Subsystem
  Divide : Product  Inputs=*/
  Divide1 : Product  Inputs=*/
  Product1 : Product
  Product2 : Product
  Product3 : Product
  Scope1 : Scope
  Scope2 : Scope
  Subsystem1 : Subsystem
  Subsystem2 : Subsystem
  Strain : Outport
  wires:
  D(Xi)1/1(D) -> Product1/1
  Strain_0/1 -> Product1/2
  Xi/1 -> Subsystem1/1(Xi), [Xi]
  Subsystem1/1(Omega) -> Scope1/1, Product2/1
  Xi_0/1 -> Subsystem2/1(Xi), D(Xi)1/1(Xi)
  Subsystem2/1(Omega) -> Product3/1
  Xi_s_0/1 -> Product3/2
  Add/1 -> Divide/1
  Sigma_0/1 -> Add1/2
  Sigma/1 -> Add1/1
  Add1/1 -> Add/1
  Xi_s/1 -> Product2/2
  Product1/1 -> Add/2
  Product3/1 -> Add/3
  Product2/1 -> Add/4, Divide1/1
  [Xi] -> D(Xi)2/1(Xi)
  D(Xi)2/1(D) -> Divide/2
  Divide/1 -> Strain/1
  [Xi] -> D(Xi)3/1(Xi)
  D(Xi)3/1(D) -> Divide1/2
  Divide1/1 -> Scope2/1

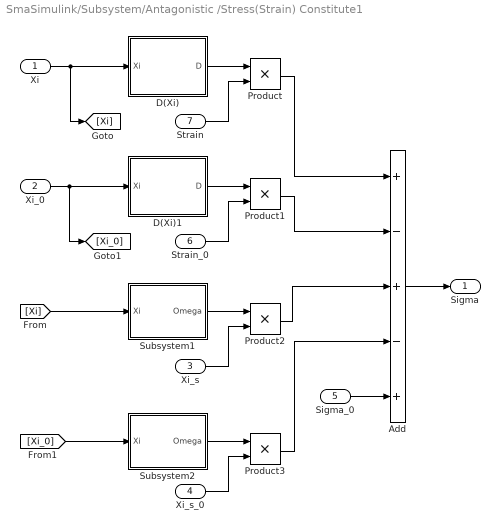
== system SmaSimulink/Subsystem/Antagonistic /Stress(Strain) Constitute1 ==
  Xi : Inport
  Xi_0 : Inport  Port=2
  Xi_s : Inport  Port=3
  Xi_s_0 : Inport  Port=4
  Sigma_0 : Inport  Port=5
  Strain_0 : Inport  Port=6
  Strain : Inport  Port=7
  Add : Sum  Inputs=+-+-+
  D(Xi) : Subsystem
  D(Xi)1 : Subsystem
  Product{,1..3} (4 alike) : Product
  Subsystem1 : Subsystem
  Subsystem2 : Subsystem
  Sigma : Outport
  wires:
  Xi/1 -> [Xi], D(Xi)/1(Xi)
  D(Xi)/1(D) -> Product/1
  Strain/1 -> Product/2
  Xi_0/1 -> [Xi_0], D(Xi)1/1(Xi)
  D(Xi)1/1(D) -> Product1/1
  Strain_0/1 -> Product1/2
  [Xi] -> Subsystem1/1(Xi)
  Subsystem1/1(Omega) -> Product2/1
  Xi_s/1 -> Product2/2
  [Xi_0] -> Subsystem2/1(Xi)
  Subsystem2/1(Omega) -> Product3/1
  Xi_s_0/1 -> Product3/2
  Product/1 -> Add/1
  Product1/1 -> Add/2
  Product2/1 -> Add/3
  Product3/1 -> Add/4
  Sigma_0/1 -> Add/5
  Add/1 -> Sigma/1

== system SmaSimulink/Subsystem/Antagonistic /Subsystem3 ==
  Temp : Inport
  Xi_s_in : Inport  Port=2
  Xi_t_in : Inport  Port=3
  Xi_n : Inport  Port=4
  Sigma : Inport  Port=5
  Af > T > As1 : Subsystem
  Demux : Demux  Outputs=3
  Memory : Memory
  Mux : Mux  Inputs=3
  Mux2 : Mux  Inputs=3
  Range check : Subsystem
  Xi_out : Outport
  Xi_s_out : Outport  Port=2
  Xi_t_out : Outport  Port=3
  wires:
  Af > T > As1/2(Xi_t_out) -> Mux/2
  Af > T > As1/3(Xi_out) -> Mux/3
  Sigma/1 -> Memory/1, Af > T > As1/5(Sigma)
  Temp/1 -> Range check/1(T), Af > T > As1/1(Temp)
  Xi_n/1 -> Mux2/3, Af > T > As1/4(Xi_n)
  Xi_s_in/1 -> Mux2/1, Af > T > As1/2(Xi_s_in)
  Xi_t_in/1 -> Mux2/2, Af > T > As1/3(Xi_t_in)
  Af > T > As1/1(Xi_s_out) -> Mux/1
  Demux/1 -> Xi_s_out/1
  Demux/2 -> Xi_t_out/1
  Demux/3 -> Xi_out/1
  Mux/1 -> Range check/2(Xis_new)
  Mux2/1 -> Range check/3(Xis_old)
  Range check/1(Out1) -> Demux/1
  Memory/1 -> Range check/4(Stress)

== system SmaSimulink/Subsystem/Antagonistic /T < Mf2 ==
  Xi_s_in : Inport
  Sigma : Inport  Port=2
  Add : Sum  Inputs=-+
  Constant3 : Constant  Value=0
  Constant4 : Constant
  Constant5 : Constant
  Switch : Switch  Criteria=u2 > Threshold  Threshold=cSs
  Switch1 : Switch  Criteria=u2 > Threshold  Threshold=cSf
  T < Mf SigmaCritS < T < SigmaCritF : Subsystem
  Xi_s_out : Outport
  "Xi_t_out " : Outport  Port=2
  wires:
  Constant3/1 -> Switch/3
  Sigma/1 -> Switch/2, Switch1/2, T < Mf SigmaCritS < T < SigmaCritF/2(Sigma)
  Switch/1 -> Switch1/3
  T < Mf SigmaCritS < T < SigmaCritF/1(Xi_t_out) -> Switch/1
  Xi_s_in/1 -> T < Mf SigmaCritS < T < SigmaCritF/1(Xi_s_in)
  Constant4/1 -> Add/2
  Switch1/1 -> Xi_s_out/1, Add/1
  Constant5/1 -> Switch1/1
  Add/1 -> "Xi_t_out "/1

== system SmaSimulink/Subsystem/Mf < T < Ms Sigma < SigmaCritS/[(1-x)//2] ==
  In : Inport
  Add1 : Sum  Inputs=+-
  Constant1 : Constant
  Constant3 : Constant  Value=2
  Divide1 : Product  Inputs=*/
  Out : Outport
  wires:
  Constant3/1 -> Divide1/2
  Divide1/1 -> Out/1
  Constant1/1 -> Add1/1
  In/1 -> Add1/2
  Add1/1 -> Divide1/1

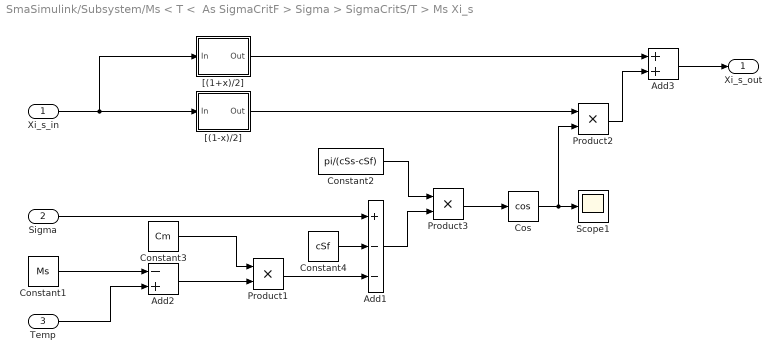
== system SmaSimulink/Subsystem/Ms < T <  As SigmaCritF > Sigma > SigmaCritS/T > Ms Xi_s ==
  Xi_s_in : Inport
  Sigma : Inport  Port=2
  Temp : Inport  Port=3
  Add1 : Sum  Inputs=+--
  Add2 : Sum  Inputs=-+
  Add3 : Sum
  Constant1 : Constant  Value=Ms
  Constant2 : Constant  Value=pi/(cSs-cSf)
  Constant3 : Constant  Value=Cm
  Constant4 : Constant  Value=cSf
  Cos : Trigonometry  Operator=cos
  Product1 : Product
  Product2 : Product
  Product3 : Product
  Scope1 : Scope
  "[(1+x)/2]" : Subsystem
  "[(1-x)/2]" : Subsystem
  Xi_s_out : Outport
  wires:
  Constant4/1 -> Add1/2
  Product1/1 -> Add1/3
  Xi_s_in/1 -> "[(1+x)/2]"/1(In), "[(1-x)/2]"/1(In)
  Add2/1 -> Product1/2
  "[(1+x)/2]"/1(Out) -> Add3/1
  Temp/1 -> Add2/2
  Product2/1 -> Add3/2
  Constant3/1 -> Product1/1
  "[(1-x)/2]"/1(Out) -> Product2/1
  Add3/1 -> Xi_s_out/1
  Constant1/1 -> Add2/1
  Sigma/1 -> Add1/1
  Add1/1 -> Product3/2
  Constant2/1 -> Product3/1
  Product3/1 -> Cos/1
  Cos/1 -> Product2/2, Scope1/1

== system SmaSimulink/Subsystem/Ms < T <  As SigmaCritF > Sigma > SigmaCritS/T > Ms Xi_t ==
  Xi_t_in : Inport
  Xi_s_in : Inport  Port=2
  Xi_s_out : Inport  Port=3
  Add1 : Sum  Inputs=+-
  Add2 : Sum  Inputs=+-
  Add3 : Sum  Inputs=-+
  Constant3 : Constant
  Divide : Product  Inputs=*/
  Product2 : Product
  Xi_t_out : Outport
  wires:
  Product2/1 -> Add1/2
  Add3/1 -> Product2/2
  Xi_s_out/1 -> Add3/2
  Xi_t_in/1 -> Divide/1, Add1/1
  Xi_s_in/1 -> Add3/1, Add2/2
  Add2/1 -> Divide/2
  Constant3/1 -> Add2/1
  Divide/1 -> Product2/1
  Add1/1 -> Xi_t_out/1

== system SmaSimulink/Subsystem/Strain(Stress) Constitute/D(Xi)1 ==
  Xi : Inport
  Add : Sum
  Constant : Constant  Value=Dm-Da
  Constant1 : Constant  Value=Da
  Product : Product
  D : Outport
  wires:
  Xi/1 -> Product/2
  Product/1 -> Add/1
  Constant1/1 -> Add/2
  Constant/1 -> Product/1
  Add/1 -> D/1

== system SmaSimulink/Subsystem/Strain(Stress) Constitute/D(Xi)2 ==
  Xi : Inport
  Add : Sum
  Constant : Constant  Value=Dm-Da
  Constant1 : Constant  Value=Da
  Product : Product
  D : Outport
  wires:
  Xi/1 -> Product/2
  Product/1 -> Add/1
  Constant1/1 -> Add/2
  Constant/1 -> Product/1
  Add/1 -> D/1

== system SmaSimulink/Subsystem/Strain(Stress) Constitute/Subsystem1 ==
  Xi : Inport
  Constant : Constant  Value=-rEmax
  Product : Product
  Subsystem1 : Subsystem
  Omega : Outport
  wires:
  Product/1 -> Omega/1
  Subsystem1/1(D) -> Product/1
  Constant/1 -> Product/2
  Xi/1 -> Subsystem1/1(Xi)

== system SmaSimulink/Subsystem/Strain(Stress) Constitute/Subsystem2 ==
  Xi : Inport
  Constant : Constant  Value=-rEmax
  Product : Product
  Subsystem1 : Subsystem
  Omega : Outport
  wires:
  Product/1 -> Omega/1
  Subsystem1/1(D) -> Product/1
  Constant/1 -> Product/2
  Xi/1 -> Subsystem1/1(Xi)

== system SmaSimulink/Subsystem/Strain(Stress) Constitute1/D(Xi)1 ==
  Xi : Inport
  Add : Sum
  Constant : Constant  Value=Dm-Da
  Constant1 : Constant  Value=Da
  Product : Product
  D : Outport
  wires:
  Xi/1 -> Product/2
  Product/1 -> Add/1
  Constant1/1 -> Add/2
  Constant/1 -> Product/1
  Add/1 -> D/1

== system SmaSimulink/Subsystem/Strain(Stress) Constitute1/D(Xi)2 ==
  Xi : Inport
  Add : Sum
  Constant : Constant  Value=Dm-Da
  Constant1 : Constant  Value=Da
  Product : Product
  D : Outport
  wires:
  Xi/1 -> Product/2
  Product/1 -> Add/1
  Constant1/1 -> Add/2
  Constant/1 -> Product/1
  Add/1 -> D/1

== system SmaSimulink/Subsystem/Strain(Stress) Constitute1/D(Xi)3 ==
  Xi : Inport
  Add : Sum
  Constant : Constant  Value=Dm-Da
  Constant1 : Constant  Value=Da
  Product : Product
  D : Outport
  wires:
  Xi/1 -> Product/2
  Product/1 -> Add/1
  Constant1/1 -> Add/2
  Constant/1 -> Product/1
  Add/1 -> D/1

== system SmaSimulink/Subsystem/Strain(Stress) Constitute1/Subsystem1 ==
  Xi : Inport
  Constant : Constant  Value=-rEmax
  Product : Product
  Subsystem1 : Subsystem
  Omega : Outport
  wires:
  Product/1 -> Omega/1
  Subsystem1/1(D) -> Product/1
  Constant/1 -> Product/2
  Xi/1 -> Subsystem1/1(Xi)

== system SmaSimulink/Subsystem/Strain(Stress) Constitute1/Subsystem2 ==
  Xi : Inport
  Constant : Constant  Value=-rEmax
  Product : Product
  Subsystem1 : Subsystem
  Omega : Outport
  wires:
  Product/1 -> Omega/1
  Subsystem1/1(D) -> Product/1
  Constant/1 -> Product/2
  Xi/1 -> Subsystem1/1(Xi)

== system SmaSimulink/Subsystem/Stress(Strain) Constitute/D(Xi) ==
  Xi : Inport
  Add : Sum
  Constant : Constant  Value=Dm-Da
  Constant1 : Constant  Value=Da
  Product : Product
  D : Outport
  wires:
  Xi/1 -> Product/2
  Product/1 -> Add/1
  Constant1/1 -> Add/2
  Constant/1 -> Product/1
  Add/1 -> D/1

== system SmaSimulink/Subsystem/Stress(Strain) Constitute/D(Xi)1 ==
  Xi : Inport
  Add : Sum
  Constant : Constant  Value=Dm-Da
  Constant1 : Constant  Value=Da
  Product : Product
  D : Outport
  wires:
  Xi/1 -> Product/2
  Product/1 -> Add/1
  Constant1/1 -> Add/2
  Constant/1 -> Product/1
  Add/1 -> D/1

== system SmaSimulink/Subsystem/Stress(Strain) Constitute/Subsystem1 ==
  Xi : Inport
  Constant : Constant  Value=-rEmax
  Product : Product
  Subsystem1 : Subsystem
  Omega : Outport
  wires:
  Product/1 -> Omega/1
  Subsystem1/1(D) -> Product/1
  Constant/1 -> Product/2
  Xi/1 -> Subsystem1/1(Xi)

== system SmaSimulink/Subsystem/Stress(Strain) Constitute/Subsystem2 ==
  Xi : Inport
  Constant : Constant  Value=-rEmax
  Product : Product
  Subsystem1 : Subsystem
  Omega : Outport
  wires:
  Product/1 -> Omega/1
  Subsystem1/1(D) -> Product/1
  Constant/1 -> Product/2
  Xi/1 -> Subsystem1/1(Xi)

== system SmaSimulink/Subsystem/Stress(Strain) Constitute1/D(Xi) ==
  Xi : Inport
  Add : Sum
  Constant : Constant  Value=Dm-Da
  Constant1 : Constant  Value=Da
  Product : Product
  D : Outport
  wires:
  Xi/1 -> Product/2
  Product/1 -> Add/1
  Constant1/1 -> Add/2
  Constant/1 -> Product/1
  Add/1 -> D/1

== system SmaSimulink/Subsystem/Stress(Strain) Constitute1/D(Xi)1 ==
  Xi : Inport
  Add : Sum
  Constant : Constant  Value=Dm-Da
  Constant1 : Constant  Value=Da
  Product : Product
  D : Outport
  wires:
  Xi/1 -> Product/2
  Product/1 -> Add/1
  Constant1/1 -> Add/2
  Constant/1 -> Product/1
  Add/1 -> D/1

== system SmaSimulink/Subsystem/Stress(Strain) Constitute1/Subsystem1 ==
  Xi : Inport
  Constant : Constant  Value=-rEmax
  Product : Product
  Subsystem1 : Subsystem
  Omega : Outport
  wires:
  Product/1 -> Omega/1
  Subsystem1/1(D) -> Product/1
  Constant/1 -> Product/2
  Xi/1 -> Subsystem1/1(Xi)

== system SmaSimulink/Subsystem/Stress(Strain) Constitute1/Subsystem2 ==
  Xi : Inport
  Constant : Constant  Value=-rEmax
  Product : Product
  Subsystem1 : Subsystem
  Omega : Outport
  wires:
  Product/1 -> Omega/1
  Subsystem1/1(D) -> Product/1
  Constant/1 -> Product/2
  Xi/1 -> Subsystem1/1(Xi)

== system SmaSimulink/Subsystem/Stress(Strain) Constitute2/D(Xi) ==
  Xi : Inport
  Add : Sum
  Constant : Constant  Value=Dm-Da
  Constant1 : Constant  Value=Da
  Product : Product
  D : Outport
  wires:
  Xi/1 -> Product/2
  Product/1 -> Add/1
  Constant1/1 -> Add/2
  Constant/1 -> Product/1
  Add/1 -> D/1

== system SmaSimulink/Subsystem/Stress(Strain) Constitute2/D(Xi)1 ==
  Xi : Inport
  Add : Sum
  Constant : Constant  Value=Dm-Da
  Constant1 : Constant  Value=Da
  Product : Product
  D : Outport
  wires:
  Xi/1 -> Product/2
  Product/1 -> Add/1
  Constant1/1 -> Add/2
  Constant/1 -> Product/1
  Add/1 -> D/1

== system SmaSimulink/Subsystem/Stress(Strain) Constitute2/Subsystem1 ==
  Xi : Inport
  Constant : Constant  Value=-rEmax
  Product : Product
  Subsystem1 : Subsystem
  Omega : Outport
  wires:
  Product/1 -> Omega/1
  Subsystem1/1(D) -> Product/1
  Constant/1 -> Product/2
  Xi/1 -> Subsystem1/1(Xi)

== system SmaSimulink/Subsystem/Stress(Strain) Constitute2/Subsystem2 ==
  Xi : Inport
  Constant : Constant  Value=-rEmax
  Product : Product
  Subsystem1 : Subsystem
  Omega : Outport
  wires:
  Product/1 -> Omega/1
  Subsystem1/1(D) -> Product/1
  Constant/1 -> Product/2
  Xi/1 -> Subsystem1/1(Xi)

== system SmaSimulink/Subsystem/Subsystem/Subsystem1 ==
  Xi : Inport
  Add : Sum
  Constant : Constant  Value=Dm-Da
  Constant1 : Constant  Value=Da
  Product : Product
  D : Outport
  wires:
  Xi/1 -> Product/2
  Product/1 -> Add/1
  Constant1/1 -> Add/2
  Constant/1 -> Product/1
  Add/1 -> D/1

== system SmaSimulink/Subsystem/Subsystem1/Af > T > As1 ==
  Temp : Inport
  Xi_s_in : Inport  Port=2
  Xi_t_in : Inport  Port=3
  Xi_n : Inport  Port=4
  Sigma : Inport  Port=5
  "T > As Xi " : Subsystem
  T > As Xi_s : Subsystem
  T > As Xi_t : Subsystem
  Xi_s_out : Outport
  Xi_t_out : Outport  Port=2
  Xi_out : Outport  Port=3
  wires:
  Sigma/1 -> "T > As Xi "/3("Sigma ")
  "T > As Xi "/1(Xi_out) -> T > As Xi_s/3(Xi_out), T > As Xi_t/3(Xi_out), Xi_out/1
  Xi_s_in/1 -> T > As Xi_s/1("Xi_s_in ")
  Xi_n/1 -> "T > As Xi "/1(Xi_in), T > As Xi_t/2(Xi_in), T > As Xi_s/2(Xi_in)
  T > As Xi_s/1(Xi_s_out) -> Xi_s_out/1
  Temp/1 -> "T > As Xi "/2(T)
  Xi_t_in/1 -> T > As Xi_t/1("Xi_t_in ")
  T > As Xi_t/1(Xi_t_out) -> Xi_t_out/1

== system SmaSimulink/Subsystem/Subsystem1/Range check ==
  T : Inport
  Xis_new : Inport  Port=2
  Xis_old : Inport  Port=3
  Stress : Inport  Port=4
  Add : Sum  Inputs=-+
  Constant1 : Constant  Value=Ca
  Constant3 : Constant  Value=[0 0 0]
  Divide : Product  Inputs=*/
  Switch : Switch  Criteria=u2 > Threshold  Threshold=As
  Switch1 : Switch  Criteria=u2 > Threshold  Threshold=Af
  Out1 : Outport
  wires:
  Switch/1 -> Switch1/3
  Constant3/1 -> Switch1/1
  Xis_old/1 -> Switch/3
  T/1 -> Add/2
  Xis_new/1 -> Switch/1
  Switch1/1 -> Out1/1
  Add/1 -> Switch/2, Switch1/2
  Stress/1 -> Divide/1
  Constant1/1 -> Divide/2
  Divide/1 -> Add/1

== system SmaSimulink/Subsystem/Subsystem2/Af > T > As1 ==
  Temp : Inport
  Xi_s_in : Inport  Port=2
  Xi_t_in : Inport  Port=3
  Xi_n : Inport  Port=4
  Sigma : Inport  Port=5
  "T > As Xi " : Subsystem
  T > As Xi_s : Subsystem
  T > As Xi_t : Subsystem
  Xi_s_out : Outport
  Xi_t_out : Outport  Port=2
  Xi_out : Outport  Port=3
  wires:
  Sigma/1 -> "T > As Xi "/3("Sigma ")
  "T > As Xi "/1(Xi_out) -> T > As Xi_s/3(Xi_out), T > As Xi_t/3(Xi_out), Xi_out/1
  Xi_s_in/1 -> T > As Xi_s/1("Xi_s_in ")
  Xi_n/1 -> "T > As Xi "/1(Xi_in), T > As Xi_t/2(Xi_in), T > As Xi_s/2(Xi_in)
  T > As Xi_s/1(Xi_s_out) -> Xi_s_out/1
  Temp/1 -> "T > As Xi "/2(T)
  Xi_t_in/1 -> T > As Xi_t/1("Xi_t_in ")
  T > As Xi_t/1(Xi_t_out) -> Xi_t_out/1

== system SmaSimulink/Subsystem/Subsystem2/Range check ==
  T : Inport
  Xis_new : Inport  Port=2
  Xis_old : Inport  Port=3
  Stress : Inport  Port=4
  Add : Sum  Inputs=-+
  Constant1 : Constant  Value=Ca
  Constant3 : Constant  Value=[0 0 0]
  Divide : Product  Inputs=*/
  Switch : Switch  Criteria=u2 > Threshold  Threshold=As
  Switch1 : Switch  Criteria=u2 > Threshold  Threshold=Af
  Out1 : Outport
  wires:
  Switch/1 -> Switch1/3
  Constant3/1 -> Switch1/1
  Xis_old/1 -> Switch/3
  T/1 -> Add/2
  Xis_new/1 -> Switch/1
  Switch1/1 -> Out1/1
  Add/1 -> Switch/2, Switch1/2
  Stress/1 -> Divide/1
  Constant1/1 -> Divide/2
  Divide/1 -> Add/1

== system SmaSimulink/Subsystem/T < Mf/T < Mf SigmaCritS < T < SigmaCritF ==
  Xi_s_in : Inport
  Sigma : Inport  Port=2
  Add1 : Sum  Inputs=+-
  Add3 : Sum
  Constant1 : Constant  Value=cSf
  Constant2 : Constant  Value=pi/(cSs-cSf)
  Cos : Trigonometry  Operator=cos
  Product2 : Product
  Product3 : Product
  "[(1+x)/2]" : Subsystem
  "[(1-x)/2]" : Subsystem
  Xi_t_out : Outport
  wires:
  Cos/1 -> Product2/2
  Product2/1 -> Add3/2
  Add1/1 -> Product3/2
  Sigma/1 -> Add1/1
  Add3/1 -> Xi_t_out/1
  Xi_s_in/1 -> "[(1+x)/2]"/1(In), "[(1-x)/2]"/1(In)
  Product3/1 -> Cos/1
  "[(1+x)/2]"/1(Out) -> Add3/1
  "[(1-x)/2]"/1(Out) -> Product2/1
  Constant2/1 -> Product3/1
  Constant1/1 -> Add1/2

== system SmaSimulink/Subsystem/T < Mf SigmaCritS < T < SigmaCritF/[(1+x)//2] ==
  In : Inport
  Add1 : Sum
  Constant1 : Constant
  Constant3 : Constant  Value=2
  Divide1 : Product  Inputs=*/
  Out : Outport
  wires:
  Constant3/1 -> Divide1/2
  Divide1/1 -> Out/1
  Constant1/1 -> Add1/1
  In/1 -> Add1/2
  Add1/1 -> Divide1/1

== system SmaSimulink/Subsystem/T < Mf SigmaCritS < T < SigmaCritF/[(1-x)//2] ==
  In : Inport
  Add1 : Sum  Inputs=+-
  Constant1 : Constant
  Constant3 : Constant  Value=2
  Divide1 : Product  Inputs=*/
  Out : Outport
  wires:
  Constant3/1 -> Divide1/2
  Divide1/1 -> Out/1
  Constant1/1 -> Add1/1
  In/1 -> Add1/2
  Add1/1 -> Divide1/1

== system SmaSimulink/Subsystem/T < Mf1/T < Mf SigmaCritS < T < SigmaCritF ==
  Xi_s_in : Inport
  Sigma : Inport  Port=2
  Add1 : Sum  Inputs=+-
  Add3 : Sum
  Constant1 : Constant  Value=cSf
  Constant2 : Constant  Value=pi/(cSs-cSf)
  Cos : Trigonometry  Operator=cos
  Product2 : Product
  Product3 : Product
  "[(1+x)/2]" : Subsystem
  "[(1-x)/2]" : Subsystem
  Xi_t_out : Outport
  wires:
  Cos/1 -> Product2/2
  Product2/1 -> Add3/2
  Add1/1 -> Product3/2
  Sigma/1 -> Add1/1
  Add3/1 -> Xi_t_out/1
  Xi_s_in/1 -> "[(1+x)/2]"/1(In), "[(1-x)/2]"/1(In)
  Product3/1 -> Cos/1
  "[(1+x)/2]"/1(Out) -> Add3/1
  "[(1-x)/2]"/1(Out) -> Product2/1
  Constant2/1 -> Product3/1
  Constant1/1 -> Add1/2

== system SmaSimulink/Subsystem/T < Mf2/T < Mf SigmaCritS < T < SigmaCritF ==
  Xi_s_in : Inport
  Sigma : Inport  Port=2
  Add1 : Sum  Inputs=+-
  Add3 : Sum
  Constant1 : Constant  Value=cSf
  Constant2 : Constant  Value=pi/(cSs-cSf)
  Cos : Trigonometry  Operator=cos
  Product2 : Product
  Product3 : Product
  "[(1+x)/2]" : Subsystem
  "[(1-x)/2]" : Subsystem
  Xi_t_out : Outport
  wires:
  Cos/1 -> Product2/2
  Product2/1 -> Add3/2
  Add1/1 -> Product3/2
  Sigma/1 -> Add1/1
  Add3/1 -> Xi_t_out/1
  Xi_s_in/1 -> "[(1+x)/2]"/1(In), "[(1-x)/2]"/1(In)
  Product3/1 -> Cos/1
  "[(1+x)/2]"/1(Out) -> Add3/1
  "[(1-x)/2]"/1(Out) -> Product2/1
  Constant2/1 -> Product3/1
  Constant1/1 -> Add1/2

== system SmaSimulink/Subsystem/T > As/Af > T > As1 ==
  Temp : Inport
  Xi_s_in : Inport  Port=2
  Xi_t_in : Inport  Port=3
  Xi_n : Inport  Port=4
  Sigma : Inport  Port=5
  "T > As Xi " : Subsystem
  T > As Xi_s : Subsystem
  T > As Xi_t : Subsystem
  Xi_s_out : Outport
  Xi_t_out : Outport  Port=2
  Xi_out : Outport  Port=3
  wires:
  Sigma/1 -> "T > As Xi "/3("Sigma ")
  "T > As Xi "/1(Xi_out) -> T > As Xi_s/3(Xi_out), T > As Xi_t/3(Xi_out), Xi_out/1
  Xi_s_in/1 -> T > As Xi_s/1("Xi_s_in ")
  Xi_n/1 -> "T > As Xi "/1(Xi_in), T > As Xi_t/2(Xi_in), T > As Xi_s/2(Xi_in)
  T > As Xi_s/1(Xi_s_out) -> Xi_s_out/1
  Temp/1 -> "T > As Xi "/2(T)
  Xi_t_in/1 -> T > As Xi_t/1("Xi_t_in ")
  T > As Xi_t/1(Xi_t_out) -> Xi_t_out/1

== system SmaSimulink/Subsystem/Antagonistic /Strain(Stress) Constitute1/D(Xi)1 ==
  Xi : Inport
  Add : Sum
  Constant : Constant  Value=Dm-Da
  Constant1 : Constant  Value=Da
  Product : Product
  D : Outport
  wires:
  Xi/1 -> Product/2
  Product/1 -> Add/1
  Constant1/1 -> Add/2
  Constant/1 -> Product/1
  Add/1 -> D/1

== system SmaSimulink/Subsystem/Antagonistic /Strain(Stress) Constitute1/D(Xi)2 ==
  Xi : Inport
  Add : Sum
  Constant : Constant  Value=Dm-Da
  Constant1 : Constant  Value=Da
  Product : Product
  D : Outport
  wires:
  Xi/1 -> Product/2
  Product/1 -> Add/1
  Constant1/1 -> Add/2
  Constant/1 -> Product/1
  Add/1 -> D/1

== system SmaSimulink/Subsystem/Antagonistic /Strain(Stress) Constitute1/D(Xi)3 ==
  Xi : Inport
  Add : Sum
  Constant : Constant  Value=Dm-Da
  Constant1 : Constant  Value=Da
  Product : Product
  D : Outport
  wires:
  Xi/1 -> Product/2
  Product/1 -> Add/1
  Constant1/1 -> Add/2
  Constant/1 -> Product/1
  Add/1 -> D/1

== system SmaSimulink/Subsystem/Antagonistic /Strain(Stress) Constitute1/Subsystem1 ==
  Xi : Inport
  Constant : Constant  Value=-rEmax
  Product : Product
  Subsystem1 : Subsystem
  Omega : Outport
  wires:
  Product/1 -> Omega/1
  Subsystem1/1(D) -> Product/1
  Constant/1 -> Product/2
  Xi/1 -> Subsystem1/1(Xi)

== system SmaSimulink/Subsystem/Antagonistic /Strain(Stress) Constitute1/Subsystem2 ==
  Xi : Inport
  Constant : Constant  Value=-rEmax
  Product : Product
  Subsystem1 : Subsystem
  Omega : Outport
  wires:
  Product/1 -> Omega/1
  Subsystem1/1(D) -> Product/1
  Constant/1 -> Product/2
  Xi/1 -> Subsystem1/1(Xi)

== system SmaSimulink/Subsystem/Antagonistic /Stress(Strain) Constitute1/D(Xi) ==
  Xi : Inport
  Add : Sum
  Constant : Constant  Value=Dm-Da
  Constant1 : Constant  Value=Da
  Product : Product
  D : Outport
  wires:
  Xi/1 -> Product/2
  Product/1 -> Add/1
  Constant1/1 -> Add/2
  Constant/1 -> Product/1
  Add/1 -> D/1

== system SmaSimulink/Subsystem/Antagonistic /Stress(Strain) Constitute1/D(Xi)1 ==
  Xi : Inport
  Add : Sum
  Constant : Constant  Value=Dm-Da
  Constant1 : Constant  Value=Da
  Product : Product
  D : Outport
  wires:
  Xi/1 -> Product/2
  Product/1 -> Add/1
  Constant1/1 -> Add/2
  Constant/1 -> Product/1
  Add/1 -> D/1

== system SmaSimulink/Subsystem/Antagonistic /Stress(Strain) Constitute1/Subsystem1 ==
  Xi : Inport
  Constant : Constant  Value=-rEmax
  Product : Product
  Subsystem1 : Subsystem
  Omega : Outport
  wires:
  Product/1 -> Omega/1
  Subsystem1/1(D) -> Product/1
  Constant/1 -> Product/2
  Xi/1 -> Subsystem1/1(Xi)

== system SmaSimulink/Subsystem/Antagonistic /Stress(Strain) Constitute1/Subsystem2 ==
  Xi : Inport
  Constant : Constant  Value=-rEmax
  Product : Product
  Subsystem1 : Subsystem
  Omega : Outport
  wires:
  Product/1 -> Omega/1
  Subsystem1/1(D) -> Product/1
  Constant/1 -> Product/2
  Xi/1 -> Subsystem1/1(Xi)

== system SmaSimulink/Subsystem/Antagonistic /Subsystem3/Af > T > As1 ==
  Temp : Inport
  Xi_s_in : Inport  Port=2
  Xi_t_in : Inport  Port=3
  Xi_n : Inport  Port=4
  Sigma : Inport  Port=5
  "T > As Xi " : Subsystem
  T > As Xi_s : Subsystem
  T > As Xi_t : Subsystem
  Xi_s_out : Outport
  Xi_t_out : Outport  Port=2
  Xi_out : Outport  Port=3
  wires:
  Sigma/1 -> "T > As Xi "/3("Sigma ")
  "T > As Xi "/1(Xi_out) -> T > As Xi_s/3(Xi_out), T > As Xi_t/3(Xi_out), Xi_out/1
  Xi_s_in/1 -> T > As Xi_s/1("Xi_s_in ")
  Xi_n/1 -> "T > As Xi "/1(Xi_in), T > As Xi_t/2(Xi_in), T > As Xi_s/2(Xi_in)
  T > As Xi_s/1(Xi_s_out) -> Xi_s_out/1
  Temp/1 -> "T > As Xi "/2(T)
  Xi_t_in/1 -> T > As Xi_t/1("Xi_t_in ")
  T > As Xi_t/1(Xi_t_out) -> Xi_t_out/1

== system SmaSimulink/Subsystem/Antagonistic /Subsystem3/Range check ==
  T : Inport
  Xis_new : Inport  Port=2
  Xis_old : Inport  Port=3
  Stress : Inport  Port=4
  Add : Sum  Inputs=-+
  Constant1 : Constant  Value=Ca
  Constant3 : Constant  Value=[0 0 0]
  Divide : Product  Inputs=*/
  Switch : Switch  Criteria=u2 > Threshold  Threshold=As
  Switch1 : Switch  Criteria=u2 > Threshold  Threshold=Af
  Out1 : Outport
  wires:
  Switch/1 -> Switch1/3
  Constant3/1 -> Switch1/1
  Xis_old/1 -> Switch/3
  T/1 -> Add/2
  Xis_new/1 -> Switch/1
  Switch1/1 -> Out1/1
  Add/1 -> Switch/2, Switch1/2
  Stress/1 -> Divide/1
  Constant1/1 -> Divide/2
  Divide/1 -> Add/1
